simulink model "Squelette_DSPBuilder_FrameGenerator"  (R2016a)
settings: Solver=FixedStepDiscrete  StartTime=0.0  StopTime=2e-3  RelTol=1e-3
InitFcn:
  | %% DSPBuilder Start
  | alt_dspbuilder_update_model(bdroot)
  | %% DSPBuilder End
libraries: allblocks_alteradspbuilder2 x174
settings Model: Creator=rhev2401  LastModifiedBy=cous2509
settings DataIOCC: LimitDataPoints=on  SaveFormat=Array  SignalLoggingSaveFormat=ModelDataLogs
settings DebuggingCC: SolverPrmCheckMsg=warning  MultiTaskDSMMsg=warning  MultiTaskCondExecSysMsg=none
settings HardwareCC: ProdBitPerPointer=32  ProdLargestAtomicFloat=None  ProdIntDivRoundTo=Undefined  ProdEndianess=Unspecified  ProdWordSize=32  ProdHWDeviceType=32-bit Generic
settings ModelReferenceCC: PropagateSignalLabelsOutOfModel=off
settings ConfigComp: CovModelRefEnable=Off  CovSFcnEnable=off

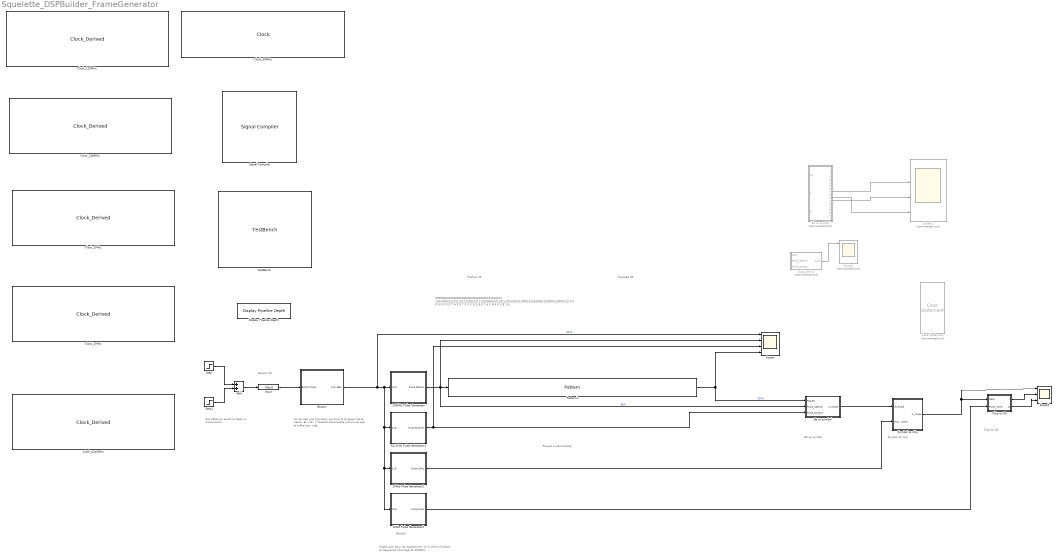
== system Squelette_DSPBuilder_FrameGenerator ==
  note: Simulates an event to begin a transmission
  note: Payload 80
  note: Prefixe 40
  note: 0000000000000000000000000000000011100101 10010000111011111111001101110100000101101110010100110001010100001010000110000110
      | 0 0 0 0 0 0 0 0 7 A 9 0 7 F F C E 2 8 6 7 A C 8 A 0 5 8 1 6
  note: Bouton 01
  note: On se crée une impulsion qui dure la longueur de la trame.
      |
      | En vrai, il faudrait transmettre jusqu'à ce que le buffer soit vide...
  note: Paquet à transmettre
  note: Bitclock
  note: Notez que, pour ce programme, on a choisi d'utiliser la fréquence d'horloge de 100MHz.
  note: Bit to symbol
  note: Symbol to chip
  note: Chip to I/Q
  1MHz Pulse Generator2 : Subsystem
  250kHz Pulse Generator : Subsystem
  2MHz Pulse Generator2 : Subsystem
  62.5kHz Pulse Generator1 : Subsystem
  Add : Sum
  Bit to symbol : Subsystem
  "Bit to symbol " : Subsystem  Commented=on
  Bouton : Subsystem
  Case Statement : allblocks_alteradspbuilder2/Case Statement  Commented=on  numOutputs=16  case_expression=0,1,2,3,4,5,6,7,8,9,10,11,12,13,14,15  formatted_case_expression=0000,0001,0010,0011,0100,0101,0110,0111,1000,1001,1010,1011,1100,1101,1110,1111  BusType=Unsigned Integer  bwl=4  bwr=0  pipeline=off  pipeline_display=0  hasDefault=off
  Chip to I/Q : Subsystem
  Clock_100MHz : allblocks_alteradspbuilder2/Clock_Derived  ClockNumerator=1  ClockDenominator=2  ResetLatency=0  ResetRegisterCascadeDepth=0  SimulationStartCycle=5  PhaseOffset=0  Reset=aclr_100MHz  ResetType=Active Low  Export=off
  Clock_125MHz : allblocks_alteradspbuilder2/Clock_Derived  ClockNumerator=10  ClockDenominator=25  ResetLatency=0  ResetRegisterCascadeDepth=0  SimulationStartCycle=5  PhaseOffset=0  Reset=aclr_125MHz  ResetType=Active Low  Export=off
  Clock_1MHz : allblocks_alteradspbuilder2/Clock_Derived  ClockNumerator=50  ClockDenominator=1  ResetLatency=0  ResetRegisterCascadeDepth=0  SimulationStartCycle=5  PhaseOffset=0  Reset=aclr_1MHz  ResetType=Active Low  Export=off
  Clock_2MHz : allblocks_alteradspbuilder2/Clock_Derived  ClockNumerator=25  ClockDenominator=1  ResetLatency=0  ResetRegisterCascadeDepth=0  SimulationStartCycle=5  PhaseOffset=0  Reset=aclr_2MHz  ResetType=Active Low  Export=off
  Clock_50MHz : allblocks_alteradspbuilder2/Clock  ClockPeriod=20  ClockPeriodUnit=ns  SampleTime=20e-9  ResetLatency=0  ResetRegisterCascadeDepth=0  SimulationStartCycle=5  PhaseOffset=0  Reset=aclr  ResetType=Active Low  Export=off
  Clock_62p5MHz : allblocks_alteradspbuilder2/Clock_Derived  ClockNumerator=800  ClockDenominator=1  ResetLatency=0  ResetRegisterCascadeDepth=0  SimulationStartCycle=5  PhaseOffset=0  Reset=aclr_62p5MHz  ResetType=Active Low  Export=off
  Display Pipeline Depth : allblocks_alteradspbuilder2/Display Pipeline Depth  DisplayLatencyOnBlocks=on
  Input : allblocks_alteradspbuilder2/Input  iofile=U:\S6\Projet\Squelette_FrameGenerator\tb_Squelette_DSPBuilder_FrameGenerator\Squelette%5FDSPBuilder%5FFrameGenerator_Input.salt  BusType=Single Bit  bwl=1  bwr=0  SpecifyClock=on  clock=Clock_100MHz  PORTTYPE=Input  externalType=Inferred  allowFloatingPointOverride=on  logOutputs=off
  Pattern1 : allblocks_alteradspbuilder2/Pattern  Sequence=<binary blob, 120 chars, not shown>  SpecifyClock=off  clock=Clock_250kHz  use_ena=on  use_sclr=off
  Scope : Scope  NumInputPorts=4
  Scope1 : Scope  Commented=on  NumInputPorts=4
  Scope2 : Scope  NumInputPorts=3
  Scope4 : Scope  Commented=on  NumInputPorts=4
  Signal Compiler : allblocks_alteradspbuilder2/Signal Compiler  DeviceFamily=Cyclone V  DeviceName=AUTO  DisableEarlyHDLGeneration=off  EnableSignalTap=off  SignalTapDepth=128  UseBoardBlock=off  StpUseDefaultClock=on  StpClock=Clock_50MHz  ExportDir=C:\Users\pivd2501\Documents  MAX10_ProgrammingMode=Internal Flash (SDM) Single Boot
  Step : Step  Time=100e-6  Before=1  After=0  SampleTime=1/100e06  VectorParams1D=off
  Step1 : Step  Time=200e-6  SampleTime=1/100e06  VectorParams1D=off
  Subsystem2 : Subsystem  Commented=on
  Symbol to chip : Subsystem
  TestBench : allblocks_alteradspbuilder2/TestBench  enable=on  advancedMode=on  modelSimGui=on  maxDisplayErrors=1000  mismatchErrorLevel=Error  simdatafile=U:\S6\Projet\Squelette_FrameGenerator\tb_Squelette_DSPBuilder_FrameGenerator\Squelette_DSPBuilder_FrameGenerator.simdata.tcl
  wires:
  Add/1 -> Input/1
  Step1/1 -> Add/2
  Step/1 -> Add/1
  250kHz Pulse Generator/1(Pulse 250kHz) -> Scope/2, Bit to symbol/2(Pulse_250kHz), Pattern1/1  "ENA"
  Bouton/1(CLR 480u) -> 1MHz Pulse Generator2/1(CLR), 2MHz Pulse Generator2/1(CLR), 62.5kHz Pulse Generator1/1(CLR), 250kHz Pulse Generator/1(CLR), Scope/1  "SCLR"
  Input/1 -> Bouton/1(Button Press)
  "Bit to symbol "/8(7) -> Scope1/2
  "Bit to symbol "/11(A) -> Scope1/3
  "Bit to symbol "/10(9) -> Scope1/4
  Pattern1/1 -> Scope/4, Bit to symbol/1(Paquet)  "DATA"
  62.5kHz Pulse Generator1/1(Pulse 62.5kHz) -> Bit to symbol/3(Pulse_62.5kHz), Scope/3
  Subsystem2/1(Out1) -> Scope4/1
  Bit to symbol/1(symbole) -> Symbol to chip/1(Symbole)
  2MHz Pulse Generator2/1(Pulse 2MHz) -> Symbol to chip/2("Pulse_2MHz ")
  Symbol to chip/1(O_Chips) -> Chip to I/Q/1(Data), Scope2/1
  1MHz Pulse Generator2/1(Pulse 1MHz) -> Chip to I/Q/2(Pulse_1MHz)
  Chip to I/Q/1("I ") -> Scope2/2
  Chip to I/Q/2(Q) -> Scope2/3

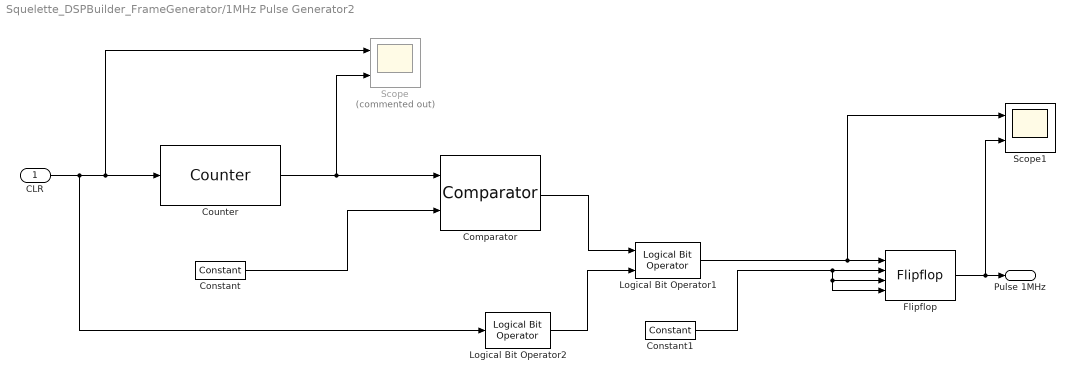
== system Squelette_DSPBuilder_FrameGenerator/1MHz Pulse Generator2 ==
  CLR : Inport
  Comparator : allblocks_alteradspbuilder2/Comparator  direction=a == b  pipeline_display=0  allowFloatingPointOverride=on  logOutputs=off  logFile=U:\S6\Projet\Squelette_FrameGenerator\tb_Squelette_DSPBuilder_FrameGenerator\Squelette%5FDSPBuilder%5FFrameGenerator_1MHz+Pulse+Generator2_Comparator.fixedpointlog
  Constant : allblocks_alteradspbuilder2/Constant  mask_cst=0  BusType=Unsigned Integer  bwl=1  bwr=0  roundMode=Truncate  satMode=Wrap  SpecifyClock=off  allowFloatingPointOverride=on  logOutputs=off  logFile=U:\S6\Projet\Squelette_FrameGenerator\tb_Squelette_DSPBuilder_FrameGenerator\Squelette%5FDSPBuilder%5FFrameGenerator_1MHz+Pulse+Generator2_Constant.fixedpointlog
  Constant1 : allblocks_alteradspbuilder2/Constant  mask_cst=1  BusType=Unsigned Integer  bwl=1  bwr=0  roundMode=Truncate  satMode=Wrap  SpecifyClock=off  allowFloatingPointOverride=on  logOutputs=off  logFile=U:\S6\Projet\Squelette_FrameGenerator\tb_Squelette_DSPBuilder_FrameGenerator\Squelette%5FDSPBuilder%5FFrameGenerator_1MHz+Pulse+Generator2_Constant1.fixedpointlog
  Counter : allblocks_alteradspbuilder2/Counter  BusType=Unsigned Integer  bwl=10  bwr=0  use_modulo=on  modulo=100  SpecifyClock=off  direction=Increment  use_sload=off  use_sset=off  svalue=1  use_clk_ena=off  use_ena=off  use_sclr=on  pipeline_display=1
  Flipflop : allblocks_alteradspbuilder2/Flipflop  mode=DFFE  BusType=Single Bit  bwl=2  bwr=2  pipeline_display=1
  Logical Bit Operator1 : allblocks_alteradspbuilder2/Logical Bit Operator  LogicalOperator=AND  user_inputs=2  pipeline_display=0
  Logical Bit Operator2 : allblocks_alteradspbuilder2/Logical Bit Operator  LogicalOperator=NOT  user_inputs=2  pipeline_display=0
  Scope : Scope  Commented=on  NumInputPorts=2
  Scope1 : Scope  NumInputPorts=2
  Pulse 1MHz : Outport
  wires:
  Logical Bit Operator1/1 -> Flipflop/1, Scope1/1
  Constant1/1 -> Flipflop/2, Flipflop/3, Flipflop/4
  Flipflop/1 -> Pulse 1MHz/1, Scope1/2
  Comparator/1 -> Logical Bit Operator1/1
  Logical Bit Operator2/1 -> Logical Bit Operator1/2
  CLR/1 -> Counter/1, Scope/1, Logical Bit Operator2/1
  Constant/1 -> Comparator/2
  Counter/1 -> Comparator/1, Scope/2

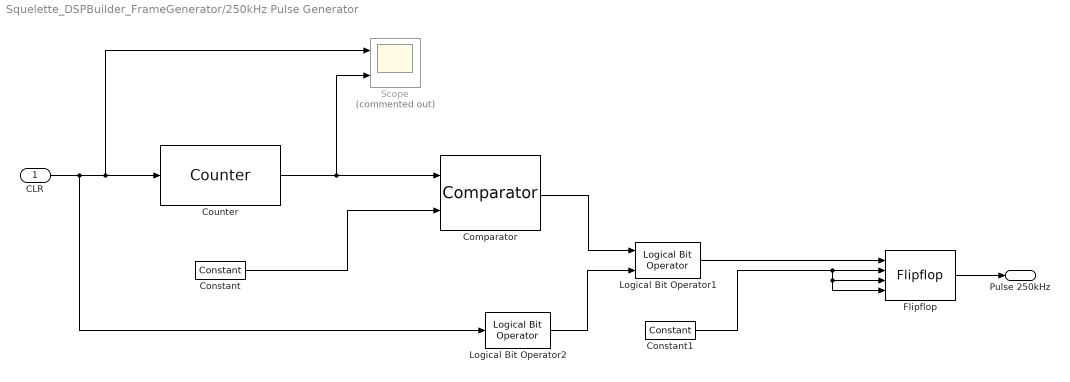
== system Squelette_DSPBuilder_FrameGenerator/250kHz Pulse Generator ==
  CLR : Inport
  Comparator : allblocks_alteradspbuilder2/Comparator  direction=a == b  pipeline_display=0  allowFloatingPointOverride=on  logOutputs=off  logFile=U:\S6\Projet\Squelette_FrameGenerator\tb_Squelette_DSPBuilder_FrameGenerator\Squelette%5FDSPBuilder%5FFrameGenerator_250kHz+Pulse+Generator_Comparator.fixedpointlog
  Constant : allblocks_alteradspbuilder2/Constant  mask_cst=0  BusType=Unsigned Integer  bwl=1  bwr=0  roundMode=Truncate  satMode=Wrap  SpecifyClock=off  allowFloatingPointOverride=on  logOutputs=off  logFile=U:\S6\Projet\Squelette_FrameGenerator\tb_Squelette_DSPBuilder_FrameGenerator\Squelette%5FDSPBuilder%5FFrameGenerator_250kHz+Pulse+Generator_Constant.fixedpointlog
  Constant1 : allblocks_alteradspbuilder2/Constant  mask_cst=1  BusType=Unsigned Integer  bwl=1  bwr=0  roundMode=Truncate  satMode=Wrap  SpecifyClock=off  allowFloatingPointOverride=on  logOutputs=off  logFile=U:\S6\Projet\Squelette_FrameGenerator\tb_Squelette_DSPBuilder_FrameGenerator\Squelette%5FDSPBuilder%5FFrameGenerator_250kHz+Pulse+Generator_Constant1.fixedpointlog
  Counter : allblocks_alteradspbuilder2/Counter  BusType=Unsigned Integer  bwl=10  bwr=0  use_modulo=on  modulo=400  SpecifyClock=off  direction=Increment  use_sload=off  use_sset=off  svalue=1  use_clk_ena=off  use_ena=off  use_sclr=on  pipeline_display=1
  Flipflop : allblocks_alteradspbuilder2/Flipflop  mode=DFFE  BusType=Single Bit  bwl=2  bwr=2  pipeline_display=1
  Logical Bit Operator1 : allblocks_alteradspbuilder2/Logical Bit Operator  LogicalOperator=AND  user_inputs=2  pipeline_display=0
  Logical Bit Operator2 : allblocks_alteradspbuilder2/Logical Bit Operator  LogicalOperator=NOT  user_inputs=2  pipeline_display=0
  Scope : Scope  Commented=on  NumInputPorts=2
  Pulse 250kHz : Outport
  wires:
  Counter/1 -> Scope/2, Comparator/1
  Constant/1 -> Comparator/2
  CLR/1 -> Logical Bit Operator2/1, Scope/1, Counter/1
  Logical Bit Operator2/1 -> Logical Bit Operator1/2
  Comparator/1 -> Logical Bit Operator1/1
  Flipflop/1 -> Pulse 250kHz/1
  Logical Bit Operator1/1 -> Flipflop/1
  Constant1/1 -> Flipflop/4, Flipflop/3, Flipflop/2

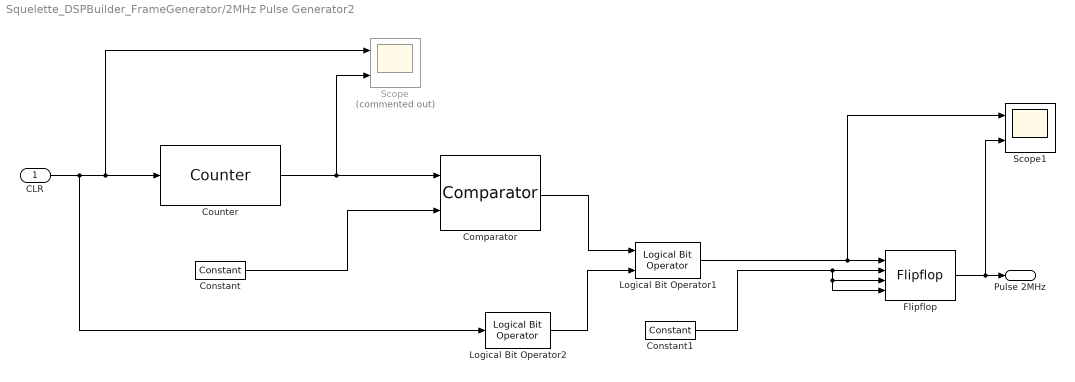
== system Squelette_DSPBuilder_FrameGenerator/2MHz Pulse Generator2 ==
  CLR : Inport
  Comparator : allblocks_alteradspbuilder2/Comparator  direction=a == b  pipeline_display=0  allowFloatingPointOverride=on  logOutputs=off  logFile=U:\S6\Projet\Squelette_FrameGenerator\tb_Squelette_DSPBuilder_FrameGenerator\Squelette%5FDSPBuilder%5FFrameGenerator_2MHz+Pulse+Generator2_Comparator.fixedpointlog
  Constant : allblocks_alteradspbuilder2/Constant  mask_cst=0  BusType=Unsigned Integer  bwl=1  bwr=0  roundMode=Truncate  satMode=Wrap  SpecifyClock=off  allowFloatingPointOverride=on  logOutputs=off  logFile=U:\S6\Projet\Squelette_FrameGenerator\tb_Squelette_DSPBuilder_FrameGenerator\Squelette%5FDSPBuilder%5FFrameGenerator_2MHz+Pulse+Generator2_Constant.fixedpointlog
  Constant1 : allblocks_alteradspbuilder2/Constant  mask_cst=1  BusType=Unsigned Integer  bwl=1  bwr=0  roundMode=Truncate  satMode=Wrap  SpecifyClock=off  allowFloatingPointOverride=on  logOutputs=off  logFile=U:\S6\Projet\Squelette_FrameGenerator\tb_Squelette_DSPBuilder_FrameGenerator\Squelette%5FDSPBuilder%5FFrameGenerator_2MHz+Pulse+Generator2_Constant1.fixedpointlog
  Counter : allblocks_alteradspbuilder2/Counter  BusType=Unsigned Integer  bwl=8  bwr=0  use_modulo=on  modulo=50  SpecifyClock=off  direction=Increment  use_sload=off  use_sset=off  svalue=1  use_clk_ena=off  use_ena=off  use_sclr=on  pipeline_display=1
  Flipflop : allblocks_alteradspbuilder2/Flipflop  mode=DFFE  BusType=Single Bit  bwl=2  bwr=2  pipeline_display=1
  Logical Bit Operator1 : allblocks_alteradspbuilder2/Logical Bit Operator  LogicalOperator=AND  user_inputs=2  pipeline_display=0
  Logical Bit Operator2 : allblocks_alteradspbuilder2/Logical Bit Operator  LogicalOperator=NOT  user_inputs=2  pipeline_display=0
  Scope : Scope  Commented=on  NumInputPorts=2
  Scope1 : Scope  NumInputPorts=2
  Pulse 2MHz : Outport
  wires:
  Counter/1 -> Scope/2, Comparator/1
  Constant/1 -> Comparator/2
  CLR/1 -> Logical Bit Operator2/1, Scope/1, Counter/1
  Logical Bit Operator2/1 -> Logical Bit Operator1/2
  Comparator/1 -> Logical Bit Operator1/1
  Flipflop/1 -> Scope1/2, Pulse 2MHz/1
  Constant1/1 -> Flipflop/4, Flipflop/3, Flipflop/2
  Logical Bit Operator1/1 -> Scope1/1, Flipflop/1

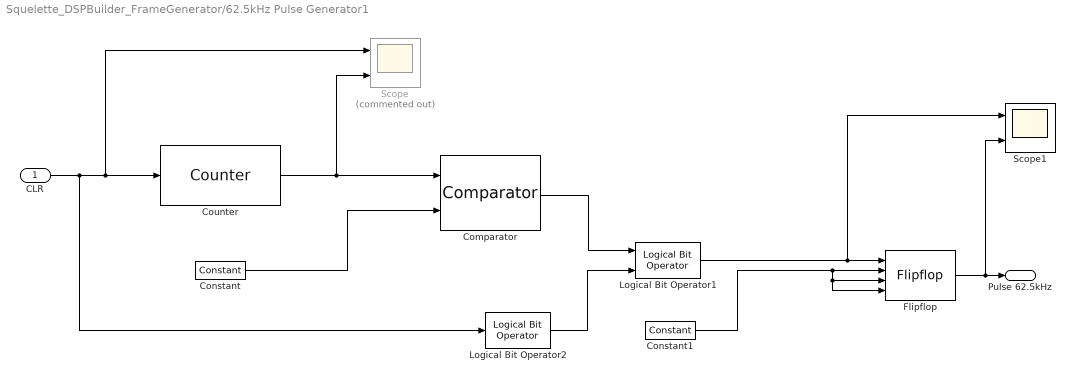
== system Squelette_DSPBuilder_FrameGenerator/62.5kHz Pulse Generator1 ==
  CLR : Inport
  Comparator : allblocks_alteradspbuilder2/Comparator  direction=a == b  pipeline_display=0  allowFloatingPointOverride=on  logOutputs=off  logFile=U:\S6\Projet\Squelette_FrameGenerator\tb_Squelette_DSPBuilder_FrameGenerator\Squelette%5FDSPBuilder%5FFrameGenerator_62.5kHz+Pulse+Generator1_Comparator.fixedpointlog
  Constant : allblocks_alteradspbuilder2/Constant  mask_cst=0  BusType=Unsigned Integer  bwl=1  bwr=0  roundMode=Truncate  satMode=Wrap  SpecifyClock=off  allowFloatingPointOverride=on  logOutputs=off  logFile=U:\S6\Projet\Squelette_FrameGenerator\tb_Squelette_DSPBuilder_FrameGenerator\Squelette%5FDSPBuilder%5FFrameGenerator_62.5kHz+Pulse+Generator1_Constant.fixedpointlog
  Constant1 : allblocks_alteradspbuilder2/Constant  mask_cst=1  BusType=Unsigned Integer  bwl=1  bwr=0  roundMode=Truncate  satMode=Wrap  SpecifyClock=off  allowFloatingPointOverride=on  logOutputs=off  logFile=U:\S6\Projet\Squelette_FrameGenerator\tb_Squelette_DSPBuilder_FrameGenerator\Squelette%5FDSPBuilder%5FFrameGenerator_62.5kHz+Pulse+Generator1_Constant1.fixedpointlog
  Counter : allblocks_alteradspbuilder2/Counter  BusType=Unsigned Integer  bwl=12  bwr=0  use_modulo=on  modulo=1600  SpecifyClock=off  direction=Increment  use_sload=off  use_sset=off  svalue=1  use_clk_ena=off  use_ena=off  use_sclr=on  pipeline_display=1
  Flipflop : allblocks_alteradspbuilder2/Flipflop  mode=DFFE  BusType=Single Bit  bwl=2  bwr=2  pipeline_display=1
  Logical Bit Operator1 : allblocks_alteradspbuilder2/Logical Bit Operator  LogicalOperator=AND  user_inputs=2  pipeline_display=0
  Logical Bit Operator2 : allblocks_alteradspbuilder2/Logical Bit Operator  LogicalOperator=NOT  user_inputs=2  pipeline_display=0
  Scope : Scope  Commented=on  NumInputPorts=2
  Scope1 : Scope  NumInputPorts=2
  Pulse 62.5kHz : Outport
  wires:
  Counter/1 -> Scope/2, Comparator/1
  Constant/1 -> Comparator/2
  CLR/1 -> Logical Bit Operator2/1, Scope/1, Counter/1
  Logical Bit Operator2/1 -> Logical Bit Operator1/2
  Comparator/1 -> Logical Bit Operator1/1
  Flipflop/1 -> Scope1/2, Pulse 62.5kHz/1
  Constant1/1 -> Flipflop/4, Flipflop/3, Flipflop/2
  Logical Bit Operator1/1 -> Scope1/1, Flipflop/1

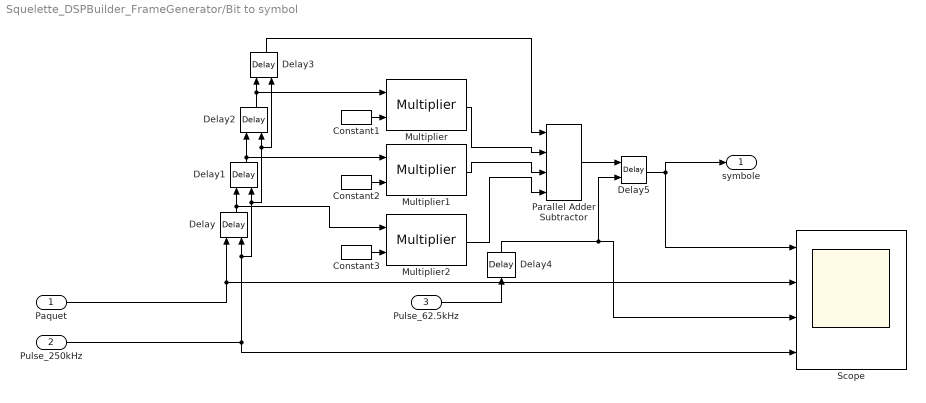
== system Squelette_DSPBuilder_FrameGenerator/Bit to symbol ==
  Paquet : Inport
  Pulse_250kHz : Inport  Port=2
  Pulse_62.5kHz : Inport  Port=3
  Constant1 : allblocks_alteradspbuilder2/Constant  mask_cst=2  BusType=Unsigned Integer  bwl=4  bwr=0  roundMode=Truncate  satMode=Wrap  SpecifyClock=off  allowFloatingPointOverride=on  logOutputs=off  logFile=U:\S6\Projet\Squelette_FrameGenerator\tb_Squelette_DSPBuilder_FrameGenerator\Squelette%5FDSPBuilder%5FFrameGenerator_Bit+to+symbol_Constant1.fixedpointlog
  Constant2 : allblocks_alteradspbuilder2/Constant  mask_cst=4  BusType=Unsigned Integer  bwl=4  bwr=0  roundMode=Truncate  satMode=Wrap  SpecifyClock=off  allowFloatingPointOverride=on  logOutputs=off  logFile=U:\S6\Projet\Squelette_FrameGenerator\tb_Squelette_DSPBuilder_FrameGenerator\Squelette%5FDSPBuilder%5FFrameGenerator_Bit+to+symbol_Constant2.fixedpointlog
  Constant3 : allblocks_alteradspbuilder2/Constant  mask_cst=8  BusType=Unsigned Integer  bwl=4  bwr=0  roundMode=Truncate  satMode=Wrap  SpecifyClock=off  allowFloatingPointOverride=on  logOutputs=off  logFile=U:\S6\Projet\Squelette_FrameGenerator\tb_Squelette_DSPBuilder_FrameGenerator\Squelette%5FDSPBuilder%5FFrameGenerator_Bit+to+symbol_Constant3.fixedpointlog
  Delay : allblocks_alteradspbuilder2/Delay  pipeline=1  pipeline_display=1  ClockPhase=1  use_ena=on  use_sclr=off  allowFloatingPointOverride=on  logOutputs=off  logFile=U:\S6\Projet\Squelette_FrameGenerator\tb_Squelette_DSPBuilder_FrameGenerator\Squelette%5FDSPBuilder%5FFrameGenerator_Bit+to+symbol_Delay.fixedpointlog  use_init=off  reset_value=1
  Delay1 : allblocks_alteradspbuilder2/Delay  pipeline=1  pipeline_display=1  ClockPhase=1  use_ena=on  use_sclr=off  allowFloatingPointOverride=on  logOutputs=off  logFile=U:\S6\Projet\Squelette_FrameGenerator\tb_Squelette_DSPBuilder_FrameGenerator\Squelette%5FDSPBuilder%5FFrameGenerator_Bit+to+symbol_Delay1.fixedpointlog  use_init=off  reset_value=1
  Delay2 : allblocks_alteradspbuilder2/Delay  pipeline=1  pipeline_display=1  ClockPhase=1  use_ena=on  use_sclr=off  allowFloatingPointOverride=on  logOutputs=off  logFile=U:\S6\Projet\Squelette_FrameGenerator\tb_Squelette_DSPBuilder_FrameGenerator\Squelette%5FDSPBuilder%5FFrameGenerator_Bit+to+symbol_Delay2.fixedpointlog  use_init=off  reset_value=1
  Delay3 : allblocks_alteradspbuilder2/Delay  pipeline=1  pipeline_display=1  ClockPhase=1  use_ena=on  use_sclr=off  allowFloatingPointOverride=on  logOutputs=off  logFile=U:\S6\Projet\Squelette_FrameGenerator\tb_Squelette_DSPBuilder_FrameGenerator\Squelette%5FDSPBuilder%5FFrameGenerator_Bit+to+symbol_Delay3.fixedpointlog  use_init=off  reset_value=1
  Delay4 : allblocks_alteradspbuilder2/Delay  pipeline=1  pipeline_display=1  ClockPhase=1  use_ena=off  use_sclr=off  allowFloatingPointOverride=on  logOutputs=off  logFile=U:\S6\Projet\Squelette_FrameGenerator\tb_Squelette_DSPBuilder_FrameGenerator\Squelette%5FDSPBuilder%5FFrameGenerator_Bit+to+symbol_Delay4.fixedpointlog  use_init=off  reset_value=1
  Delay5 : allblocks_alteradspbuilder2/Delay  pipeline=1  pipeline_display=1  ClockPhase=1  use_ena=on  use_sclr=off  allowFloatingPointOverride=on  logOutputs=off  logFile=U:\S6\Projet\Squelette_FrameGenerator\tb_Squelette_DSPBuilder_FrameGenerator\Squelette%5FDSPBuilder%5FFrameGenerator_Bit+to+symbol_Delay5.fixedpointlog  use_init=off  reset_value=1
  Multiplier : allblocks_alteradspbuilder2/Multiplier  BusType=Unsigned Integer  bwl=1  bwr=0  pipeline=0  pipeline_display=0  allowFloatingPointOverride=on  logOutputs=off  logFile=U:\S6\Projet\Squelette_FrameGenerator\tb_Squelette_DSPBuilder_FrameGenerator\Squelette%5FDSPBuilder%5FFrameGenerator_Bit+to+symbol_Multiplier.fixedpointlog  UseEqualInputWidth=off  bbwl=2  bbwr=0  FullResolution=on  OutputMsb=8  OutputLsb=0  OutputBwl=16  OutputBwr=16  UseDedicatedCircuitry=YES  use_ena=off  use_aclr=off
  Multiplier1 : allblocks_alteradspbuilder2/Multiplier  BusType=Unsigned Integer  bwl=1  bwr=0  pipeline=0  pipeline_display=0  allowFloatingPointOverride=on  logOutputs=off  logFile=U:\S6\Projet\Squelette_FrameGenerator\tb_Squelette_DSPBuilder_FrameGenerator\Squelette%5FDSPBuilder%5FFrameGenerator_Bit+to+symbol_Multiplier1.fixedpointlog  UseEqualInputWidth=off  bbwl=3  bbwr=0  FullResolution=on  OutputMsb=8  OutputLsb=0  OutputBwl=16  OutputBwr=16  UseDedicatedCircuitry=YES  use_ena=off  use_aclr=off
  Multiplier2 : allblocks_alteradspbuilder2/Multiplier  BusType=Unsigned Integer  bwl=1  bwr=0  pipeline=0  pipeline_display=0  allowFloatingPointOverride=on  logOutputs=off  logFile=U:\S6\Projet\Squelette_FrameGenerator\tb_Squelette_DSPBuilder_FrameGenerator\Squelette%5FDSPBuilder%5FFrameGenerator_Bit+to+symbol_Multiplier2.fixedpointlog  UseEqualInputWidth=off  bbwl=4  bbwr=0  FullResolution=on  OutputMsb=8  OutputLsb=0  OutputBwl=16  OutputBwr=16  UseDedicatedCircuitry=YES  use_ena=off  use_aclr=off
  Parallel Adder Subtractor : allblocks_alteradspbuilder2/Parallel Adder Subtractor  number_of_inputs=4  direction=+  use_pipeline=off  pipeline_display=0  phase_selection=1  use_ena=on  use_aclr=off  allowFloatingPointOverride=on  logOutputs=off  logFile=U:\S6\Projet\Squelette_FrameGenerator\tb_Squelette_DSPBuilder_FrameGenerator\Squelette%5FDSPBuilder%5FFrameGenerator_Bit+to+symbol_Parallel+Adder+Subtractor.fixedpointlog
  Scope : Scope  NumInputPorts=4
  symbole : Outport
  wires:
  Pulse_250kHz/1 -> Delay3/2, Delay2/2, Delay1/2, Delay/2, Scope/4
  Paquet/1 -> Delay/1, Scope/2
  Delay2/1 -> Multiplier/1, Delay3/1
  Constant1/1 -> Multiplier/2
  Delay1/1 -> Multiplier1/1, Delay2/1
  Constant2/1 -> Multiplier1/2
  Delay/1 -> Multiplier2/1, Delay1/1
  Constant3/1 -> Multiplier2/2
  Pulse_62.5kHz/1 -> Delay4/1
  Delay5/1 -> symbole/1, Scope/1
  Multiplier/1 -> Parallel Adder Subtractor/2
  Multiplier1/1 -> Parallel Adder Subtractor/3
  Multiplier2/1 -> Parallel Adder Subtractor/4
  Delay4/1 -> Scope/3, Delay5/2
  Parallel Adder Subtractor/1 -> Delay5/1
  Delay3/1 -> Parallel Adder Subtractor/1

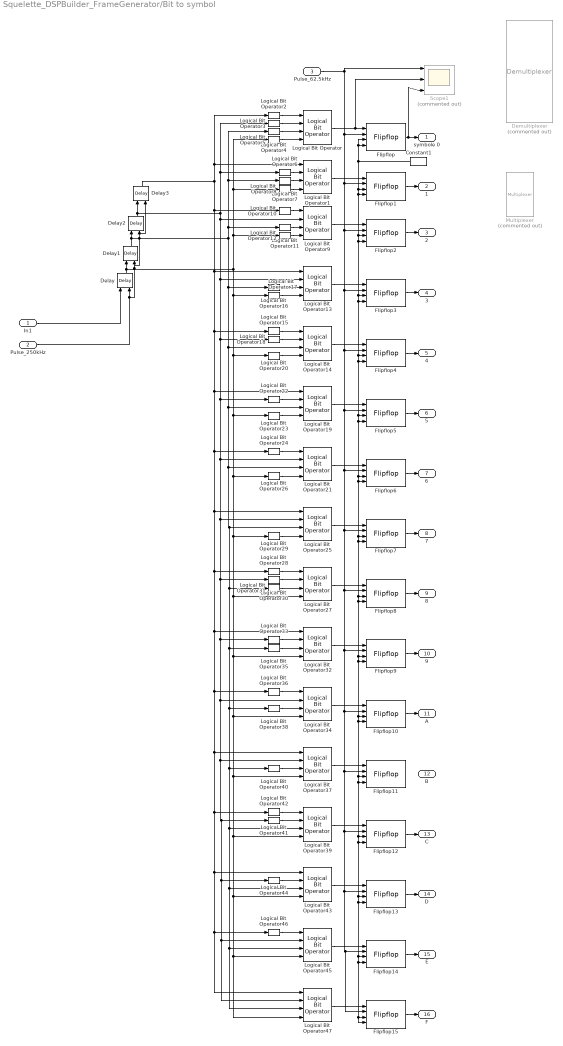
== system Squelette_DSPBuilder_FrameGenerator/Bit to symbol  ==
  In1 : Inport
  Pulse_250kHz : Inport  Port=2
  "Pulse_62.5kHz " : Inport  Port=3
  Constant1 : allblocks_alteradspbuilder2/Constant  mask_cst=1  BusType=Unsigned Integer  bwl=1  bwr=0  roundMode=Truncate  satMode=Wrap  SpecifyClock=off  allowFloatingPointOverride=on  logOutputs=off  logFile=U:\S6\Projet\Squelette_FrameGenerator\tb_Squelette_DSPBuilder_FrameGenerator\Squelette%5FDSPBuilder%5FFrameGenerator_Bit+to+symbol%0A_Constant1.fixedpointlog
  Delay : allblocks_alteradspbuilder2/Delay  pipeline=1  pipeline_display=1  ClockPhase=1  use_ena=on  use_sclr=off  allowFloatingPointOverride=on  logOutputs=off  logFile=U:\S6\Projet\Squelette_FrameGenerator\tb_Squelette_DSPBuilder_FrameGenerator\Squelette%5FDSPBuilder%5FFrameGenerator_Bit+to+symbol%0A_Delay.fixedpointlog  use_init=off  reset_value=1
  Delay1 : allblocks_alteradspbuilder2/Delay  pipeline=1  pipeline_display=1  ClockPhase=1  use_ena=on  use_sclr=off  allowFloatingPointOverride=on  logOutputs=off  logFile=U:\S6\Projet\Squelette_FrameGenerator\tb_Squelette_DSPBuilder_FrameGenerator\Squelette%5FDSPBuilder%5FFrameGenerator_Bit+to+symbol%0A_Delay1.fixedpointlog  use_init=off  reset_value=1
  Delay2 : allblocks_alteradspbuilder2/Delay  pipeline=1  pipeline_display=1  ClockPhase=1  use_ena=on  use_sclr=off  allowFloatingPointOverride=on  logOutputs=off  logFile=U:\S6\Projet\Squelette_FrameGenerator\tb_Squelette_DSPBuilder_FrameGenerator\Squelette%5FDSPBuilder%5FFrameGenerator_Bit+to+symbol%0A_Delay2.fixedpointlog  use_init=off  reset_value=1
  Delay3 : allblocks_alteradspbuilder2/Delay  pipeline=1  pipeline_display=1  ClockPhase=1  use_ena=on  use_sclr=off  allowFloatingPointOverride=on  logOutputs=off  logFile=U:\S6\Projet\Squelette_FrameGenerator\tb_Squelette_DSPBuilder_FrameGenerator\Squelette%5FDSPBuilder%5FFrameGenerator_Bit+to+symbol%0A_Delay3.fixedpointlog  use_init=off  reset_value=1
  Demultiplexer : allblocks_alteradspbuilder2/Demultiplexer  Commented=on  numOutputs=16  pipeline_display=1  use_ena=off  use_sclr=off  allowFloatingPointOverride=on  logOutputs=off  logFile=U:\S6\Projet\Squelette_FrameGenerator\tb_Squelette_DSPBuilder_FrameGenerator\Squelette%5FDSPBuilder%5FFrameGenerator_Bit+to+symbol%0A_Demultiplexer%3A%3Aq.fixedpointlog,U:\S6\Projet\Squelette_FrameGenerator\tb_Squelette_DSPBuilder_FrameGenerator\Squelette%5FDSPBuilder%5FFrameGenerator_Bit+to+symbol%0A_Demultiplexer%3A%3Aq.fixedpointlog,U:\S6\Projet\Squelette_FrameGenerator\tb_Squelette_DSPBuilder_FrameGenerator\Squelette%5FDSPBuilder%5FFrameGenerator_Bit+to+symbol%0A_Demultiplexer%3A%3Aq.fixedpointlog,U:\S6\Projet\Squelette_FrameGenerator\tb_Squelette_DSPBuilder_FrameGenerator\Squelette%5FDSPBuilder%5FFrameGenerator_Bit+to+symbol%0A_Demultiplexer%3A%3Aq.fixedpointlog,U:\S6\Projet\Squelette_FrameGenerator\tb_Squelette_DSPBuilder_FrameGenerator\Squelette%5FDSPBuilder%5FFrameGenerator_Bit+to+symbol%0A_Demultiplexer%3A%3Aq.fixedpointlog,U:\S6\Projet\Squelette_FrameGenerator\tb_Squelette_DSPBuilder_FrameGenerator\Squelette%5FDSPBuilder%5FFrameGenerator_Bit+to+symbol%0A_Demultiplexer%3A%3Aq.fixedpointlog,U:\S6\Projet\Squelette_FrameGenerator\tb_Squelette_DSPBuilder_FrameGenerator\Squelette%5FDSPBuilder%5FFrameGenerator_Bit+to+symbol%0A_Demultiplexer%3A%3Aq.fixedpointlog,U:\S6\Projet\Squelette_FrameGenerator\tb_Squelette_DSPBuilder_FrameGenerator\Squelette%5FDSPBuilder%5FFrameGenerator_Bit+to+symbol%0A_Demultiplexer%3A%3Aq.fixedpointlog,U:\S6\Projet\Squelette_FrameGenerator\tb_Squelette_DSPBuilder_FrameGenerator\Squelette%5FDSPBuilder%5FFrameGenerator_Bit+to+symbol%0A_Demultiplexer%3A%3Aq.fixedpointlog,U:\S6\Projet\Squelette_FrameGenerator\tb_Squelette_DSPBuilder_FrameGenerator\Squelette%5FDSPBuilder%5FFrameGenerator_Bit+to+symbol%0A_Demultiplexer%3A%3Aq.fixedpointlog,U:\S6\Projet\Squelette_FrameGenerator\tb_Squelette_DSPBuilder_FrameGenerator\Squelette%5FDSPBuilder%5FFrameGenerator_Bit+to+symbol%0A_Demultiplexer%3A%3Aq.fixedpointlog,U:\S6\Projet\Squelette_FrameGenerator\tb_Squelette_DSPBuilder_FrameGenerator\Squelette%5FDSPBuilder%5FFrameGenerator_Bit+to+symbol%0A_Demultiplexer%3A%3Aq.fixedpointlog,U:\S6\Projet\Squelette_FrameGenerator\tb_Squelette_DSPBuilder_FrameGenerator\Squelette%5FDSPBuilder%5FFrameGenerator_Bit+to+symbol%0A_Demultiplexer%3A%3Aq.fixedpointlog,U:\S6\Projet\Squelette_FrameGenerator\tb_Squelette_DSPBuilder_FrameGenerator\Squelette%5FDSPBuilder%5FFrameGenerator_Bit+to+symbol%0A_Demultiplexer%3A%3Aq.fixedpointlog,U:\S6\Projet\Squelette_FrameGenerator\tb_Squelette_DSPBuilder_FrameGenerator\Squelette%5FDSPBuilder%5FFrameGenerator_Bit+to+symbol%0A_Demultiplexer%3A%3Aq.fixedpointlog,U:\S6\Projet\Squelette_FrameGenerator\tb_Squelette_DSPBuilder_FrameGenerator\Squelette%5FDSPBuilder%5FFrameGenerator_Bit+to+symbol%0A_Demultiplexer%3A%3Aq.fixedpointlog,
  Flipflop{,1..15} (16 alike) : allblocks_alteradspbuilder2/Flipflop  mode=DFFE  BusType=Single Bit  bwl=2  bwr=2  pipeline_display=1
  Logical Bit Operator{,1,9,13..14,19,21,25,27,32,34,37,39,43,45,47} (16 alike) : allblocks_alteradspbuilder2/Logical Bit Operator  LogicalOperator=AND  user_inputs=4  pipeline_display=0
  Logical Bit Operator{2..8,10..12,15..18,20,22..24,26,28..31,33,35..36,38,40..42,44,46} (32 alike) : allblocks_alteradspbuilder2/Logical Bit Operator  LogicalOperator=NOT  user_inputs=2  pipeline_display=0
  Multiplexer : allblocks_alteradspbuilder2/Multiplexer  Commented=on  numInputs=6  pipeline=0  oneHot=off  pipeline_display=0  use_ena=off  use_aclr=off  allowFloatingPointOverride=on  logOutputs=off  logFile=U:\S6\Projet\Squelette_FrameGenerator\tb_Squelette_DSPBuilder_FrameGenerator\Squelette%5FDSPBuilder%5FFrameGenerator_Bit+to+symbol%0A_Multiplexer.fixedpointlog
  Scope1 : Scope  Commented=on  NumInputPorts=3
  symbole 0 : Outport
  1 : Outport  Port=2
  2 : Outport  Port=3
  3 : Outport  Port=4
  4 : Outport  Port=5
  5 : Outport  Port=6
  6 : Outport  Port=7
  7 : Outport  Port=8
  8 : Outport  Port=9
  9 : Outport  Port=10
  A : Outport  Port=11
  B : Outport  Port=12
  C : Outport  Port=13
  D : Outport  Port=14
  E : Outport  Port=15
  F : Outport  Port=16
  wires:
  In1/1 -> Delay/1
  Logical Bit Operator2/1 -> Logical Bit Operator/1
  Logical Bit Operator3/1 -> Logical Bit Operator/2
  Logical Bit Operator4/1 -> Logical Bit Operator/3
  Logical Bit Operator5/1 -> Logical Bit Operator/4
  Logical Bit Operator6/1 -> Logical Bit Operator1/2
  Logical Bit Operator7/1 -> Logical Bit Operator1/3
  Logical Bit Operator8/1 -> Logical Bit Operator1/4
  Logical Bit Operator11/1 -> Logical Bit Operator9/3
  Logical Bit Operator12/1 -> Logical Bit Operator9/4
  Logical Bit Operator10/1 -> Logical Bit Operator9/1
  Logical Bit Operator16/1 -> Logical Bit Operator13/3
  Logical Bit Operator17/1 -> Logical Bit Operator13/4
  Logical Bit Operator15/1 -> Logical Bit Operator14/1
  Logical Bit Operator18/1 -> Logical Bit Operator14/2
  Logical Bit Operator20/1 -> Logical Bit Operator14/4
  Logical Bit Operator22/1 -> Logical Bit Operator19/2
  Logical Bit Operator23/1 -> Logical Bit Operator19/4
  Logical Bit Operator24/1 -> Logical Bit Operator21/1
  Logical Bit Operator26/1 -> Logical Bit Operator21/4
  Logical Bit Operator29/1 -> Logical Bit Operator25/4
  Logical Bit Operator28/1 -> Logical Bit Operator27/1
  Logical Bit Operator30/1 -> Logical Bit Operator27/2
  Logical Bit Operator31/1 -> Logical Bit Operator27/3
  Logical Bit Operator35/1 -> Logical Bit Operator32/3
  Logical Bit Operator38/1 -> Logical Bit Operator34/3
  Logical Bit Operator33/1 -> Logical Bit Operator32/2
  Logical Bit Operator36/1 -> Logical Bit Operator34/1
  Logical Bit Operator40/1 -> Logical Bit Operator37/3
  Logical Bit Operator41/1 -> Logical Bit Operator39/2
  Logical Bit Operator42/1 -> Logical Bit Operator39/1
  Logical Bit Operator44/1 -> Logical Bit Operator43/2
  Logical Bit Operator46/1 -> Logical Bit Operator45/1
  Delay/1 -> Logical Bit Operator12/1, Logical Bit Operator5/1, Logical Bit Operator8/1, Logical Bit Operator47/4, Logical Bit Operator45/4, Logical Bit Operator43/4, Logical Bit Operator39/4, Logical Bit Operator37/4, Logical Bit Operator34/4, Logical Bit Operator32/4, Logical Bit Operator27/4, Logical Bit Operator29/1, Logical Bit Operator26/1, Logical Bit Operator23/1, Logical Bit Operator20/1, Logical Bit Operator17/1, Delay1/1
  Delay1/1 -> Delay2/1, Logical Bit Operator11/1, Logical Bit Operator4/1, Logical Bit Operator7/1, Logical Bit Operator47/3, Logical Bit Operator45/3, Logical Bit Operator43/3, Logical Bit Operator39/3, Logical Bit Operator40/1, Logical Bit Operator38/1, Logical Bit Operator35/1, Logical Bit Operator31/1, Logical Bit Operator25/3, Logical Bit Operator21/3, Logical Bit Operator19/3, Logical Bit Operator14/3, Logical Bit Operator16/1
  Delay2/1 -> Delay3/1, Logical Bit Operator3/1, Logical Bit Operator6/1, Logical Bit Operator47/2, Logical Bit Operator45/2, Logical Bit Operator44/1, Logical Bit Operator41/1, Logical Bit Operator37/2, Logical Bit Operator34/2, Logical Bit Operator33/1, Logical Bit Operator30/1, Logical Bit Operator25/2, Logical Bit Operator21/2, Logical Bit Operator22/1, Logical Bit Operator18/1, Logical Bit Operator13/2, Logical Bit Operator9/2
  Delay3/1 -> Logical Bit Operator2/1, Logical Bit Operator1/1, Logical Bit Operator32/1, Logical Bit Operator47/1, Logical Bit Operator46/1, Logical Bit Operator43/1, Logical Bit Operator42/1, Logical Bit Operator37/1, Logical Bit Operator36/1, Logical Bit Operator28/1, Logical Bit Operator25/1, Logical Bit Operator24/1, Logical Bit Operator19/1, Logical Bit Operator15/1, Logical Bit Operator13/1, Logical Bit Operator10/1
  Pulse_250kHz/1 -> Delay3/2, Delay2/2, Delay1/2, Delay/2
  Logical Bit Operator/1 -> Scope1/2, Flipflop/1
  Flipflop/1 -> Scope1/3, symbole 0/1
  Constant1/1 -> Flipflop1/3, Flipflop1/4, Flipflop15/4, Flipflop15/3, Flipflop14/4, Flipflop14/3, Flipflop13/4, Flipflop13/3, Flipflop12/4, Flipflop12/3, Flipflop11/4, Flipflop11/3, Flipflop10/4, Flipflop10/3, Flipflop9/4, Flipflop9/3, Flipflop8/4, Flipflop8/3, Flipflop7/4, Flipflop7/3, Flipflop6/4, Flipflop6/3, Flipflop5/4, Flipflop5/3, Flipflop4/4, Flipflop4/3, Flipflop3/4, Flipflop3/3, Flipflop2/4, Flipflop2/3, Flipflop/4, Flipflop/3
  Logical Bit Operator1/1 -> Flipflop1/1
  Flipflop1/1 -> 1/1
  Logical Bit Operator9/1 -> Flipflop2/1
  Flipflop2/1 -> 2/1
  Flipflop3/1 -> 3/1
  Flipflop4/1 -> 4/1
  Flipflop5/1 -> 5/1
  Flipflop6/1 -> 6/1
  Flipflop7/1 -> 7/1
  Flipflop8/1 -> 8/1
  Flipflop9/1 -> 9/1
  Flipflop10/1 -> A/1
  Flipflop12/1 -> C/1
  Flipflop13/1 -> D/1
  Flipflop14/1 -> E/1
  Flipflop15/1 -> F/1
  Logical Bit Operator13/1 -> Flipflop3/1
  Logical Bit Operator14/1 -> Flipflop4/1
  Logical Bit Operator19/1 -> Flipflop5/1
  Logical Bit Operator21/1 -> Flipflop6/1
  Logical Bit Operator25/1 -> Flipflop7/1
  Logical Bit Operator27/1 -> Flipflop8/1
  Logical Bit Operator32/1 -> Flipflop9/1
  Logical Bit Operator34/1 -> Flipflop10/1
  Logical Bit Operator37/1 -> Flipflop11/1
  Logical Bit Operator39/1 -> Flipflop12/1
  Logical Bit Operator43/1 -> Flipflop13/1
  "Pulse_62.5kHz "/1 -> Scope1/1, Flipflop1/2, Flipflop2/2, Flipflop3/2, Flipflop4/2, Flipflop6/2, Flipflop7/2, Flipflop11/2, Flipflop15/2, Flipflop14/2, Flipflop13/2, Flipflop12/2, Flipflop10/2, Flipflop9/2, Flipflop8/2, Flipflop5/2, Flipflop/2
  Logical Bit Operator45/1 -> Flipflop14/1
  Logical Bit Operator47/1 -> Flipflop15/1

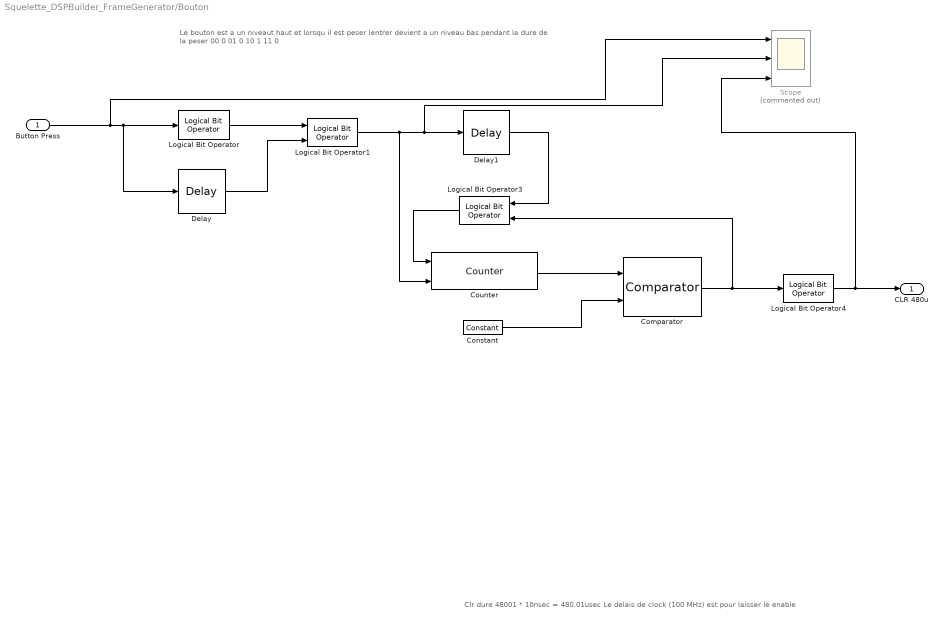
== system Squelette_DSPBuilder_FrameGenerator/Bouton ==
  note: Clr dure 48001 * 10nsec = 480.01usec Le delais de clock (100 MHz) est pour laisser le enable
  note: Le bouton est a un niveaut haut et lorsqu il est peser lentrer devient a un niveau bas pendant la dure de la peser
      |
      | 00  0
      | 01  0
      | 10  1
      | 11  0
  Button Press : Inport
  Comparator : allblocks_alteradspbuilder2/Comparator  direction=a >= b  pipeline_display=0  allowFloatingPointOverride=on  logOutputs=off  logFile=U:\S6\Projet\Squelette_FrameGenerator\tb_Squelette_DSPBuilder_FrameGenerator\Squelette%5FDSPBuilder%5FFrameGenerator_Bouton_Comparator.fixedpointlog
  Constant : allblocks_alteradspbuilder2/Constant  mask_cst=1  BusType=Unsigned Integer  bwl=8  bwr=0  roundMode=Truncate  satMode=Wrap  SpecifyClock=off  allowFloatingPointOverride=on  logOutputs=off  logFile=U:\S6\Projet\Squelette_FrameGenerator\tb_Squelette_DSPBuilder_FrameGenerator\Squelette%5FDSPBuilder%5FFrameGenerator_Bouton_Constant.fixedpointlog
  Counter : allblocks_alteradspbuilder2/Counter  BusType=Unsigned Integer  bwl=16  bwr=0  use_modulo=on  modulo=48001  SpecifyClock=off  clock=Clock_100MHz  direction=Increment  use_sload=off  use_sset=off  svalue=1  use_clk_ena=off  use_ena=on  use_sclr=on  pipeline_display=1
  Delay : allblocks_alteradspbuilder2/Delay  pipeline=1  pipeline_display=1  ClockPhase=1  use_ena=off  use_sclr=off  allowFloatingPointOverride=on  logOutputs=off  logFile=U:\S6\Projet\Squelette_FrameGenerator\tb_Squelette_DSPBuilder_FrameGenerator\Squelette%5FDSPBuilder%5FFrameGenerator_Bouton_Delay.fixedpointlog  use_init=off  reset_value=1
  Delay1 : allblocks_alteradspbuilder2/Delay  pipeline=1  pipeline_display=1  ClockPhase=1  use_ena=off  use_sclr=off  allowFloatingPointOverride=on  logOutputs=off  logFile=U:\S6\Projet\Squelette_FrameGenerator\tb_Squelette_DSPBuilder_FrameGenerator\Squelette%5FDSPBuilder%5FFrameGenerator_Bouton_Delay1.fixedpointlog  use_init=off  reset_value=1
  Logical Bit Operator : allblocks_alteradspbuilder2/Logical Bit Operator  LogicalOperator=NOT  user_inputs=2  pipeline_display=0
  Logical Bit Operator1 : allblocks_alteradspbuilder2/Logical Bit Operator  LogicalOperator=AND  user_inputs=2  pipeline_display=0
  Logical Bit Operator3 : allblocks_alteradspbuilder2/Logical Bit Operator  LogicalOperator=OR  user_inputs=2  pipeline_display=0
  Logical Bit Operator4 : allblocks_alteradspbuilder2/Logical Bit Operator  LogicalOperator=NOT  user_inputs=2  pipeline_display=0
  Scope : Scope  Commented=on  NumInputPorts=3
  CLR 480u : Outport
  wires:
  Button Press/1 -> Scope/1, Logical Bit Operator/1, Delay/1
  Logical Bit Operator/1 -> Logical Bit Operator1/1
  Logical Bit Operator1/1 -> Scope/2, Delay1/1, Counter/2
  Counter/1 -> Comparator/1
  Constant/1 -> Comparator/2
  Delay1/1 -> Logical Bit Operator3/1
  Logical Bit Operator3/1 -> Counter/1
  Comparator/1 -> Logical Bit Operator3/2, Logical Bit Operator4/1
  Delay/1 -> Logical Bit Operator1/2
  Logical Bit Operator4/1 -> Scope/3, CLR 480u/1

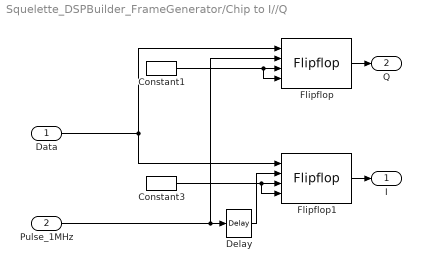
== system Squelette_DSPBuilder_FrameGenerator/Chip to I//Q ==
  Data : Inport
  Pulse_1MHz : Inport  Port=2
  Constant1 : allblocks_alteradspbuilder2/Constant  mask_cst=1  BusType=Unsigned Integer  bwl=1  bwr=0  roundMode=Truncate  satMode=Wrap  SpecifyClock=off  allowFloatingPointOverride=on  logOutputs=off  logFile=U:\S6\Projet\Squelette_FrameGenerator\tb_Squelette_DSPBuilder_FrameGenerator\Squelette%5FDSPBuilder%5FFrameGenerator_Chip+to+I__Q_Constant1.fixedpointlog
  Constant3 : allblocks_alteradspbuilder2/Constant  mask_cst=1  BusType=Unsigned Integer  bwl=1  bwr=0  roundMode=Truncate  satMode=Wrap  SpecifyClock=off  allowFloatingPointOverride=on  logOutputs=off  logFile=U:\S6\Projet\Squelette_FrameGenerator\tb_Squelette_DSPBuilder_FrameGenerator\Squelette%5FDSPBuilder%5FFrameGenerator_Chip+to+I__Q_Constant3.fixedpointlog
  Delay : allblocks_alteradspbuilder2/Delay  pipeline=1  pipeline_display=1  ClockPhase=1  use_ena=off  use_sclr=off  allowFloatingPointOverride=on  logOutputs=off  logFile=U:\S6\Projet\Squelette_FrameGenerator\tb_Squelette_DSPBuilder_FrameGenerator\Squelette%5FDSPBuilder%5FFrameGenerator_Chip+to+I__Q_Delay.fixedpointlog  use_init=off  reset_value=1
  Flipflop : allblocks_alteradspbuilder2/Flipflop  mode=DFFE  BusType=Single Bit  bwl=2  bwr=2  pipeline_display=1
  Flipflop1 : allblocks_alteradspbuilder2/Flipflop  mode=DFFE  BusType=Single Bit  bwl=2  bwr=2  pipeline_display=1
  "I " : Outport
  Q : Outport  Port=2
  wires:
  Constant3/1 -> Flipflop1/4, Flipflop1/3
  Constant1/1 -> Flipflop/4, Flipflop/3
  Flipflop1/1 -> "I "/1
  Flipflop/1 -> Q/1
  Pulse_1MHz/1 -> Delay/1, Flipflop/2
  Data/1 -> Flipflop1/1, Flipflop/1
  Delay/1 -> Flipflop1/2

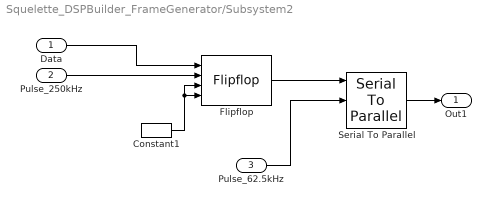
== system Squelette_DSPBuilder_FrameGenerator/Subsystem2 ==
  Data : Inport
  Pulse_250kHz : Inport  Port=2
  Pulse_62.5kHz : Inport  Port=3
  Constant1 : allblocks_alteradspbuilder2/Constant  mask_cst=1  BusType=Unsigned Integer  bwl=1  bwr=0  roundMode=Truncate  satMode=Wrap  SpecifyClock=off  allowFloatingPointOverride=on  logOutputs=off  logFile=U:\S6\Projet\Squelette_FrameGenerator\tb_Squelette_DSPBuilder_FrameGenerator\Squelette%5FDSPBuilder%5FFrameGenerator_Subsystem2_Constant1.fixedpointlog
  Flipflop : allblocks_alteradspbuilder2/Flipflop  mode=DFFE  BusType=Single Bit  bwl=2  bwr=2  pipeline_display=1
  Serial To Parallel : allblocks_alteradspbuilder2/Serial To Parallel  BusType=Unsigned Integer  bwl=4  bwr=0  msbfirsttext=LSB First  msbfirst=0  use_ena=on  use_sclr=on
  Out1 : Outport
  wires:
  Pulse_62.5kHz/1 -> Serial To Parallel/2
  Flipflop/1 -> Serial To Parallel/1
  Constant1/1 -> Flipflop/4, Flipflop/3
  Serial To Parallel/1 -> Out1/1
  Data/1 -> Flipflop/1
  Pulse_250kHz/1 -> Flipflop/2

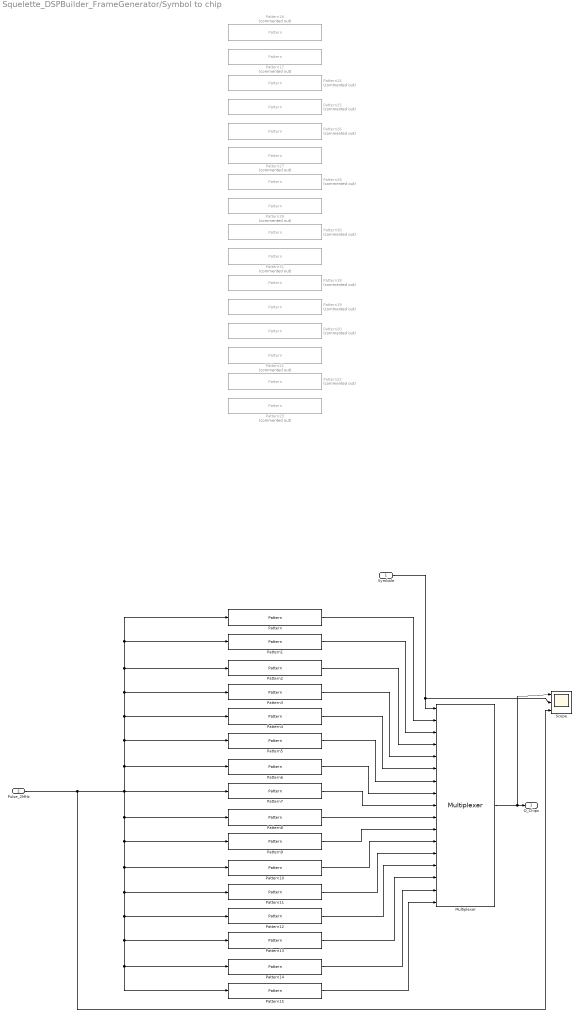
== system Squelette_DSPBuilder_FrameGenerator/Symbol to chip ==
  Symbole : Inport
  "Pulse_2MHz " : Inport  Port=2
  Multiplexer : allblocks_alteradspbuilder2/Multiplexer  numInputs=16  pipeline=0  oneHot=off  pipeline_display=0  use_ena=off  use_aclr=off  allowFloatingPointOverride=on  logOutputs=off  logFile=U:\S6\Projet\Squelette_FrameGenerator\tb_Squelette_DSPBuilder_FrameGenerator\Squelette%5FDSPBuilder%5FFrameGenerator_Symbol+to+chip_Multiplexer.fixedpointlog
  Pattern : allblocks_alteradspbuilder2/Pattern  Sequence=11011001110000110101001000101110  SpecifyClock=off  use_ena=on  use_sclr=off
  Pattern1 : allblocks_alteradspbuilder2/Pattern  Sequence=11101101100111000011010100100010  SpecifyClock=off  use_ena=on  use_sclr=off
  Pattern10 : allblocks_alteradspbuilder2/Pattern  Sequence=01111011100011001001011000000111  SpecifyClock=off  use_ena=on  use_sclr=off
  Pattern11 : allblocks_alteradspbuilder2/Pattern  Sequence=01110111101110001100100101100000  SpecifyClock=off  use_ena=on  use_sclr=off
  Pattern12 : allblocks_alteradspbuilder2/Pattern  Sequence=00000111011110111000110010010110  SpecifyClock=off  use_ena=on  use_sclr=off
  Pattern13 : allblocks_alteradspbuilder2/Pattern  Sequence=01100000011101111011100011001001  SpecifyClock=off  use_ena=on  use_sclr=off
  Pattern14 : allblocks_alteradspbuilder2/Pattern  Sequence=10010110000001110111101110001100  SpecifyClock=off  use_ena=on  use_sclr=off
  Pattern15 : allblocks_alteradspbuilder2/Pattern  Sequence=1100100101100000111011110111000  SpecifyClock=off  use_ena=on  use_sclr=off
  Pattern16 : allblocks_alteradspbuilder2/Pattern  Commented=on  Sequence=01110100010010101100001110011011  SpecifyClock=off  use_ena=on  use_sclr=off
  Pattern17 : allblocks_alteradspbuilder2/Pattern  Commented=on  Sequence=01000100101011000011100110110111  SpecifyClock=off  use_ena=on  use_sclr=off
  Pattern18 : allblocks_alteradspbuilder2/Pattern  Commented=on  Sequence=11100000011010010011000111011110  SpecifyClock=off  use_ena=on  use_sclr=off
  Pattern19 : allblocks_alteradspbuilder2/Pattern  Commented=on  Sequence=00000110100100110001110111101110  SpecifyClock=off  use_ena=on  use_sclr=off
  Pattern2 : allblocks_alteradspbuilder2/Pattern  Sequence=00101110110110011100001101010010  SpecifyClock=off  use_ena=on  use_sclr=off
  Pattern20 : allblocks_alteradspbuilder2/Pattern  Commented=on  Sequence=01101001001100011101111011100000  SpecifyClock=off  use_ena=on  use_sclr=off
  Pattern21 : allblocks_alteradspbuilder2/Pattern  Commented=on  Sequence=10010011000111011110111000000110  SpecifyClock=off  use_ena=on  use_sclr=off
  Pattern22 : allblocks_alteradspbuilder2/Pattern  Commented=on  Sequence=00110001110111101110000001101001  SpecifyClock=off  use_ena=on  use_sclr=off
  Pattern23 : allblocks_alteradspbuilder2/Pattern  Commented=on  Sequence=00011101111011100000011010010011  SpecifyClock=off  use_ena=on  use_sclr=off
  Pattern24 : allblocks_alteradspbuilder2/Pattern  Commented=on  Sequence=01001010110000111001101101110100  SpecifyClock=off  use_ena=on  use_sclr=off
  Pattern25 : allblocks_alteradspbuilder2/Pattern  Commented=on  Sequence=10101100001110011011011101000100  SpecifyClock=off  use_ena=on  use_sclr=off
  Pattern26 : allblocks_alteradspbuilder2/Pattern  Commented=on  Sequence=11000011100110110111010001001010  SpecifyClock=off  use_ena=on  use_sclr=off
  Pattern27 : allblocks_alteradspbuilder2/Pattern  Commented=on  Sequence=00111001101101110100010010101100  SpecifyClock=off  use_ena=on  use_sclr=off
  Pattern28 : allblocks_alteradspbuilder2/Pattern  Commented=on  Sequence=10011011011101000100101011000011  SpecifyClock=off  use_ena=on  use_sclr=off
  Pattern29 : allblocks_alteradspbuilder2/Pattern  Commented=on  Sequence=10110111010001001010110000111001  SpecifyClock=off  use_ena=on  use_sclr=off
  Pattern3 : allblocks_alteradspbuilder2/Pattern  Sequence=00100010111011011001110000110101  SpecifyClock=off  use_ena=on  use_sclr=off
  Pattern30 : allblocks_alteradspbuilder2/Pattern  Commented=on  Sequence=11011110111000000110100100110001  SpecifyClock=off  use_ena=on  use_sclr=off
  Pattern31 : allblocks_alteradspbuilder2/Pattern  Commented=on  Sequence=11101110000001101001001100011101  SpecifyClock=off  use_ena=on  use_sclr=off
  Pattern4 : allblocks_alteradspbuilder2/Pattern  Sequence=01010010001011101101100111000011  SpecifyClock=off  use_ena=on  use_sclr=off
  Pattern5 : allblocks_alteradspbuilder2/Pattern  Sequence=00110101001000101110110110011100  SpecifyClock=off  use_ena=on  use_sclr=off
  Pattern6 : allblocks_alteradspbuilder2/Pattern  Sequence=11000011010100100010111011011001  SpecifyClock=off  use_ena=on  use_sclr=off
  Pattern7 : allblocks_alteradspbuilder2/Pattern  Sequence=10011100001101010010001011101101  SpecifyClock=off  use_ena=on  use_sclr=off
  Pattern8 : allblocks_alteradspbuilder2/Pattern  Sequence=10001100100101100000011101111011  SpecifyClock=off  use_ena=on  use_sclr=off
  Pattern9 : allblocks_alteradspbuilder2/Pattern  Sequence=10111000110010010110000001110111  SpecifyClock=off  use_ena=on  use_sclr=off
  Scope : Scope  NumInputPorts=3
  O_Chips : Outport
  wires:
  Pattern3/1 -> Multiplexer/5
  Pattern4/1 -> Multiplexer/6
  Pattern5/1 -> Multiplexer/7
  Pattern6/1 -> Multiplexer/8
  Pattern7/1 -> Multiplexer/9
  Pattern8/1 -> Multiplexer/10
  Pattern9/1 -> Multiplexer/11
  Pattern10/1 -> Multiplexer/12
  Pattern11/1 -> Multiplexer/13
  Pattern12/1 -> Multiplexer/14
  Pattern13/1 -> Multiplexer/15
  Pattern14/1 -> Multiplexer/16
  "Pulse_2MHz "/1 -> Scope/3, Pattern8/1, Pattern9/1, Pattern10/1, Pattern11/1, Pattern12/1, Pattern13/1, Pattern14/1, Pattern15/1, Pattern7/1, Pattern6/1, Pattern5/1, Pattern4/1, Pattern3/1, Pattern2/1, Pattern1/1, Pattern/1
  Pattern15/1 -> Multiplexer/17
  Pattern/1 -> Multiplexer/2
  Pattern1/1 -> Multiplexer/3
  Pattern2/1 -> Multiplexer/4
  Multiplexer/1 -> O_Chips/1, Scope/1
  Symbole/1 -> Scope/2, Multiplexer/1
